simulink model "simu"  (R2021a)
settings: Solver=VariableStepAuto  StartTime=0.0  StopTime=200  RelTol=1e-3
libraries: dspnetwork x3, spsSinglePhaseAsynchronousMachineLib x2, spsACVoltageSourceLib x1, spsCurrentMeasurementLib x1, spsGroundLib x1, dspstat3 x1, spsVariableResistorLib x1, spsVoltageMeasurementLib x1, spspowerguiLib x1
settings Model: Creator=Hxtreme  LastModifiedBy=sofia

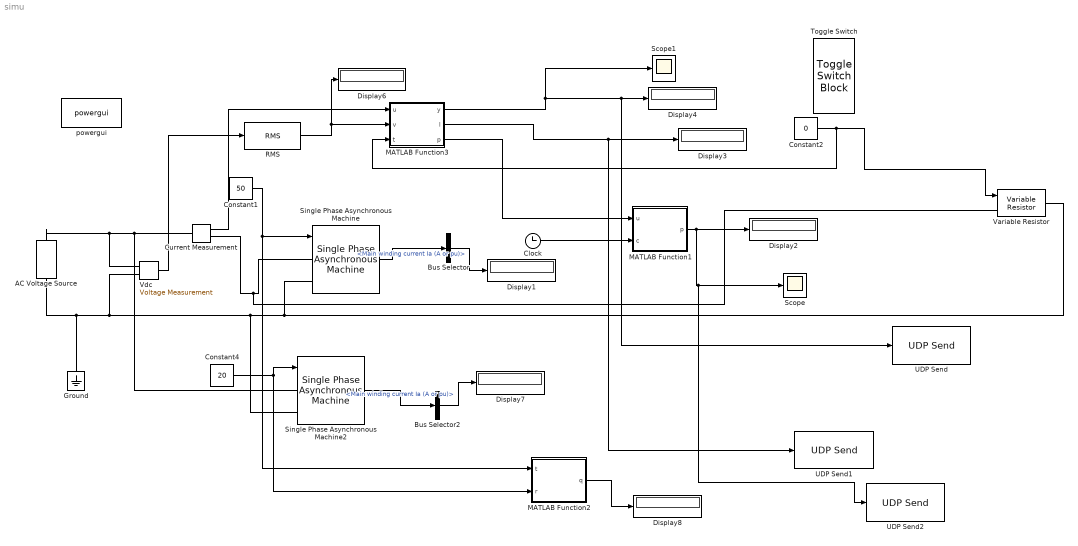
== system simu ==
  AC Voltage Source : spsACVoltageSourceLib/AC Voltage Source  Amplitude=220  Phase=0  Frequency=50  SampleTime=0  Measurements=Voltage  BusType=swing  Pref=10e3  Qref=0  Qmin=-inf  Qmax=+inf
  Bus Selector : BusSelector  OutputSignals=Stator measurements.Main winding current Ia (A or pu)
  Bus Selector2 : BusSelector  OutputSignals=Stator measurements.Main winding current Ia (A or pu)
  Clock : Clock
  Constant1 : Constant  Value=50
  Constant2 : Constant  Value=0
  Constant4 : Constant  Value=20
  Current Measurement : spsCurrentMeasurementLib/Current Measurement  PhasorSimulation=off  OutputType=Complex  PSBequivalent=0
  Display{1..4,6..8} (7 alike) : Display
  Ground : spsGroundLib/Ground  LConnTagsString=a
  MATLAB Function1 : MATLAB Function  TreatAsAtomicUnit=on
  MATLAB Function2 : MATLAB Function  TreatAsAtomicUnit=on
  MATLAB Function3 : MATLAB Function  TreatAsAtomicUnit=on
  RMS : dspstat3/RMS  run=off  directionMode=Each column  dimension=1  InputProcessing=Columns as channels (frame based)  reset_popup=None
  Scope : Scope
  Scope1 : Scope
  Single Phase Asynchronous Machine : spsSinglePhaseAsynchronousMachineLib/Single Phase Asynchronous Machine  MechanicalLoad=Torque Tm  UNITS=SI  MachineType=Split Phase  MeasurementBus=off  NominalParameters="[ .25*746  110  60]"  MainWindingStator="[2.02  7.4e-3]"  MainWindingRotor="[4.12  5.6e-3]"  MutualInductance=2000  AuxiliaryWinding="[7.14  8.5e-3]"  Mechanical="[0.0146  0  2 1.18]"  CapacitorStart="[2  254.7e-6]"  CapacitorRun="[18  21.1e-6]"  DisconnectionSpeed=75  InitialSpeed=100  DataType=SI  TsPowergui=0  TsBlock=-1
      settings: SourceProductBaseCode=PS
  Single Phase Asynchronous Machine2 : spsSinglePhaseAsynchronousMachineLib/Single Phase Asynchronous Machine  MechanicalLoad=Torque Tm  UNITS=SI  MachineType=Split Phase  MeasurementBus=off  NominalParameters="[ .25*746  110  60]"  MainWindingStator="[2.02  7.4e-3]"  MainWindingRotor="[4.12  5.6e-3]"  MutualInductance=2000  AuxiliaryWinding="[7.14  8.5e-3]"  Mechanical="[0.0146  0  2 1.18]"  CapacitorStart="[2  254.7e-6]"  CapacitorRun="[18  21.1e-6]"  DisconnectionSpeed=75  InitialSpeed=100  DataType=SI  TsPowergui=0  TsBlock=-1
      settings: SourceProductBaseCode=PS
  Toggle Switch : ToggleSwitchBlock
      settings: Values={{'Off', 'On'}, [200 0]}
  UDP Send : dspnetwork/UDP Send  remoteURL='127.0.0.1'  remotePort=5005  localURL='0.0.0.0'  localPortSource=Automatically determine  localPort=-1  sendBufferSize=8192  sampletime=-1  blockPlatform=[]  separateLengthPort=0
  UDP Send1 : dspnetwork/UDP Send  remoteURL='127.0.0.1'  remotePort=5006  localURL='0.0.0.0'  localPortSource=Automatically determine  localPort=-1  sendBufferSize=8192  sampletime=-1  blockPlatform=[]  separateLengthPort=0
  UDP Send2 : dspnetwork/UDP Send  remoteURL='127.0.0.1'  remotePort=5007  localURL='0.0.0.0'  localPortSource=Automatically determine  localPort=-1  sendBufferSize=8192  sampletime=-1  blockPlatform=[]  separateLengthPort=0
  Variable Resistor : spsVariableResistorLib/Variable Resistor  Rabsmin=1e-3
      settings: SourceProductBaseCode=PS
  "Vdc " : spsVoltageMeasurementLib/Voltage Measurement  Tag=PoWeRsYsTeMmEaSuReMeNt  PhasorSimulation=off  OutputType=Magnitude  PSBequivalent=0
  powergui : spspowerguiLib/powergui  Priority=1  SimulationMode=Discrete  SampleTime=1e-05  frequency=60  Iterations=50  frequencyindice=60  Pbase=100e6  ErrMax=1e-4  UnitsV=kV  UnitsW=MW  buscounter=0  FunctionMessages=off  echomessages=off  EnableUseOfTLC=off  CurrentSourceSwitches=off  DisableSnubberDevices=off  DisableRonSwitches=off  DisableVfSwitches=off  DisplayEquations=off  AutomaticDiscreteSolvers=off  SolverType=Tustin/Backward Euler (TBE)  Interpol=off  ExternalGateDelay=off  methode=off  Ts=100  x0status=blocks  SPID=on  SwTol=0  HookPort=off  NonlinearTolerance=1e-4  nMaxIteration=100  ContinueOnMaxIteration=off  RestoreLinks=warning  ResistiveCurrentMeasurement=off  Frange=[0:2:500]  Ylog=off  Xlog=on  ShowGrid=off  save=off  variable=ZData  structure=0  ZoomFFT=off  StartTime=0.0  cycles=1  DisplayStyle=1  fundamental=60  FreqAxis=off  MaxFrequency=1000  frequencyindicesteady=1  RmsSteady=1  display=off
  wires:
  Constant1/1 -> MATLAB Function2/1(t), Single Phase Asynchronous Machine/1
  Bus Selector/1 -> Display1/1  "<Main winding current Ia (A or pu)>"
  Current Measurement/1 -> MATLAB Function3/1(u)
  Single Phase Asynchronous Machine/1 -> Bus Selector/1
  MATLAB Function3/1(y) -> Scope1/1, UDP Send/1, Display4/1
  MATLAB Function3/3(p) -> MATLAB Function1/1(u)
  Clock/1 -> MATLAB Function1/2(c)
  MATLAB Function1/1(p) -> UDP Send2/1, Scope/1, Display2/1
  Constant2/1 -> MATLAB Function3/3(t), Variable Resistor/1
  MATLAB Function3/2(l) -> UDP Send1/1, Display3/1
  "Vdc "/1 -> RMS/1
  RMS/1 -> MATLAB Function3/2(v), Display6/1
  Bus Selector2/1 -> Display7/1  "<Main winding current Ia (A or pu)>"
  Single Phase Asynchronous Machine2/1 -> Bus Selector2/1
  MATLAB Function2/1(q) -> Display8/1
  Constant4/1 -> Single Phase Asynchronous Machine2/1, MATLAB Function2/2(r)
  connections:
  AC Voltage Source/RConn1 -- Current Measurement/LConn1 -- Single Phase Asynchronous Machine2/LConn1 -- "Vdc "/LConn1
  "Vdc "/LConn2 -- Ground/LConn1 -- AC Voltage Source/LConn1 -- Variable Resistor/RConn1 -- Single Phase Asynchronous Machine/LConn2 -- Single Phase Asynchronous Machine2/LConn2
  Current Measurement/RConn1 -- Variable Resistor/LConn1 -- Single Phase Asynchronous Machine/LConn1

== matlab function simu/MATLAB Function1 ==
  data: p output; u input; c input
function p  = fcn(u,c)
p=0
p = (u * c) / 1000000

== matlab function simu/MATLAB Function2 ==
  data: q output; t input; r input
function q  = fcn(t,r)
if t >r 
    q="Normal";
else 
    q="Over Load";
end
end

== matlab function simu/MATLAB Function3 ==
  data: u input; y output; v input; l output; p output; t input
function [y,l,p] = fcn(u,v,t)
y=0
l=0
p=0
if u<=0 
    u=-u;
end

y = (u);

y=u;
if v< 0
    l=v*-220;
else 
    l=220
end
p=y*l;

y=y*t
